simulink model "D2C_simulation_2boucles_0"  (R2013a)
settings: Solver=ode45  StartTime=0.0  StopTime=20  FixedStep=0.003  RelTol=1e-3
libraries: slctrlblks x2, simulink x2
settings Model: Creator=Propriétaire  LastModifiedBy=Propriétaire
settings DataIOCC: SignalLoggingSaveFormat=ModelDataLogs
settings OptimizationCC: ExpressionDepthLimit=2147483647
settings DebuggingCC: FcnCallInpInsideContextMsg=UseLocalSettings
settings GRTTargetCC: CombineOutputUpdateFcns=off  GRTInterface=on

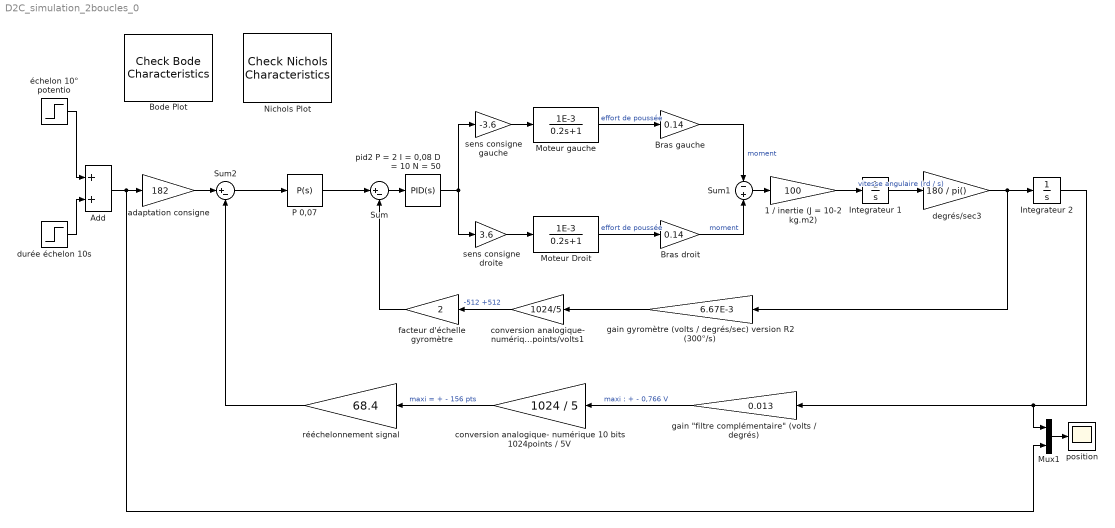
== system D2C_simulation_2boucles_0 ==
  1 / inertie (J = 10-2 kg.m2) : Gain  Gain=100
  Add : Sum
  Bode Plot : slctrlblks/Model Verification/Check Bode  Characteristics  InstantiateOnLoad=on  LinearizationIOs={'/Sum2', 1, 'in', 'on', '';'/rééchelonnement signal', 1, 'out', 'on', ''}  LinearizeAt=SnapshotTimes  SnapshotTimes=[0]  TriggerType=rising  SampleTime=auto  RateConversionMethod=zoh  PreWarpFreq=10  UseExactDelayModel=off  UseFullBlockNameLabels=off  UseBusSignalLabels=off  enabled=on  stopWhenAssertionFail=off  export=off  ViewDlgPos=[1323 39 510 390]  OpenViewOnLoad=on  LaunchViewOnOpen=on  FrequencyUnits=rad/s  MagnitudeUnits=dB  PhaseUnits=deg  TimeUnits=seconds  EnableUpperBound=off  UpperBoundFrequencies=[]  UpperBoundMagnitudes=[]  EnableLowerBound=off  LowerBoundFrequencies=[]  LowerBoundMagnitudes=[]
  Bras droit : Gain  Gain=0.14
  Bras gauche : Gain  Gain=0.14
  Integrateur 1 : Integrator
  Integrateur 2 : Integrator
  Moteur Droit : TransferFcn  Numerator=[1E-3]  Denominator=[0.2 1]
  Moteur gauche : TransferFcn  Numerator=[1E-3]  Denominator=[0.2 1]
  Mux1 : Mux  Inputs=2
  Nichols Plot : slctrlblks/Model Verification/Check Nichols Characteristics  InstantiateOnLoad=on  LinearizationIOs={'/Sum2', 1, 'in', 'on', '';'/rééchelonnement signal', 1, 'out', 'on', ''}  LinearizeAt=SnapshotTimes  SnapshotTimes=[0]  TriggerType=rising  SampleTime=auto  RateConversionMethod=zoh  PreWarpFreq=10  UseExactDelayModel=off  UseFullBlockNameLabels=off  UseBusSignalLabels=off  enabled=on  stopWhenAssertionFail=off  export=off  ViewDlgPos=[1322 516 510 390]  LaunchViewOnOpen=on  OpenViewOnLoad=on  FrequencyUnits=rad/s  MagnitudeUnits=dB  PhaseUnits=deg  TimeUnits=seconds  EnableMargins=off  GainMargin=[]  PhaseMargin=[]  EnableGainPhaseBound=off  GainPhaseBoundType={'upper'}  OLPhases=[]  OLGains=[]  EnableCLPeakGain=off  CLPeakGain=[]  FeedbackSign=-1
      settings: SaveToWorkspace=off  SaveName=sys
  P 0,07 : simulink/Continuous/PID Controller  Controller=P  TimeDomain=Continuous-time  SampleTime=1  IntegratorMethod=Forward Euler  FilterMethod=Forward Euler  Form=Parallel  P=0.07  I=5  D=0.0013  N=330  InitialConditionSource=internal  InitialConditionForIntegrator=0  InitialConditionForFilter=0  ExternalReset=none  LimitOutput=off  UpperSaturationLimit=inf  LowerSaturationLimit=-inf  LinearizeAsGain=off  AntiWindupMode=none  Kb=1  TrackingMode=off  Kt=1  PParamMin=[]  PParamMax=[]  IParamMin=[]  IParamMax=[]  DParamMin=[]  DParamMax=[]  NParamMin=[]  NParamMax=[]  KbParamMin=[]  KbParamMax=[]  KtParamMin=[]  KtParamMax=[]  POutMin=[]  POutMax=[]  IOutMin=[]  IOutMax=[]  DOutMin=[]  DOutMax=[]  NOutMin=[]  NOutMax=[]  KbOutMin=[]  KbOutMax=[]  KtOutMin=[]  KtOutMax=[]  IntegratorOutMin=[]  IntegratorOutMax=[]  FilterOutMin=[]  FilterOutMax=[]  SumOutMin=[]  SumOutMax=[]  SumI1OutMin=[]  SumI1OutMax=[]  SumI2OutMin=[]  SumI2OutMax=[]  SumI3OutMin=[]  SumI3OutMax=[]  SumDOutMin=[]  SumDOutMax=[]  SaturationOutMin=[]  SaturationOutMax=[]  IntegratorContinuousStateAttributes=''  IntegratorStateMustResolveToSignalObject=off  IntegratorRTWStateStorageClass=Auto  FilterContinuousStateAttributes=''  FilterStateMustResolveToSignalObject=off  FilterRTWStateStorageClass=Auto
  Sum : Sum  Inputs=|+-
  Sum1 : Sum  Inputs=-|+
  Sum2 : Sum  Inputs=|+-
  adaptation consigne : Gain  Gain=182
  conversion analogique- numérique points/volts1 : Gain  Gain=1024/5
  conversion analogique- numérique 10 bits 1024points / 5V : Gain  Gain=1024 / 5
  degrés/sec3 : Gain  Gain=180 / pi()
  durée échelon 10s : Step  Time=10  After=-10  SampleTime=0
  facteur d'échelle gyromètre : Gain  Gain=2
  "gain \"filtre complémentaire\" (volts / degrés)" : Gain  Gain=0.013
  gain gyromètre (volts / degrés/sec) version R2 (300°/s) : Gain  Gain=6.67E-3
  "pid2 P = 2 I = 0,08 D = 10 N = 50 " : simulink/Continuous/PID Controller  Controller=PID  TimeDomain=Continuous-time  SampleTime=1  IntegratorMethod=Forward Euler  FilterMethod=Forward Euler  Form=Parallel  P=2  I=0.08  D=10/50  N=50  InitialConditionSource=internal  InitialConditionForIntegrator=0  InitialConditionForFilter=0  ExternalReset=none  LimitOutput=off  UpperSaturationLimit=inf  LowerSaturationLimit=-inf  LinearizeAsGain=off  AntiWindupMode=none  Kb=1  TrackingMode=off  Kt=1  PParamMin=[]  PParamMax=[]  IParamMin=[]  IParamMax=[]  DParamMin=[]  DParamMax=[]  NParamMin=[]  NParamMax=[]  KbParamMin=[]  KbParamMax=[]  KtParamMin=[]  KtParamMax=[]  POutMin=[]  POutMax=[]  IOutMin=[]  IOutMax=[]  DOutMin=[]  DOutMax=[]  NOutMin=[]  NOutMax=[]  KbOutMin=[]  KbOutMax=[]  KtOutMin=[]  KtOutMax=[]  IntegratorOutMin=[]  IntegratorOutMax=[]  FilterOutMin=[]  FilterOutMax=[]  SumOutMin=[]  SumOutMax=[]  SumI1OutMin=[]  SumI1OutMax=[]  SumI2OutMin=[]  SumI2OutMax=[]  SumI3OutMin=[]  SumI3OutMax=[]  SumDOutMin=[]  SumDOutMax=[]  SaturationOutMin=[]  SaturationOutMax=[]  IntegratorContinuousStateAttributes=''  IntegratorStateMustResolveToSignalObject=off  IntegratorRTWStateStorageClass=Auto  FilterContinuousStateAttributes=''  FilterStateMustResolveToSignalObject=off  FilterRTWStateStorageClass=Auto
  position : Scope
      settings: YMin=-1  YMax=10
  rééchelonnement signal : Gain  Gain=68.4
  sens consigne droite : Gain  Gain=3.6
  sens consigne gauche : Gain  Gain=-3.6
  échelon 10° potentio : Step  Time=0  After=10  SampleTime=0
  wires:
  Moteur gauche/1 -> Bras gauche/1  "effort de poussée"
  Bras gauche/1 -> Sum1/1  "moment"
  Moteur Droit/1 -> Bras droit/1  "effort de poussée"
  Bras droit/1 -> Sum1/2  "moment"
  sens consigne gauche/1 -> Moteur gauche/1
  sens consigne droite/1 -> Moteur Droit/1
  Sum1/1 -> 1 / inertie (J = 10-2 kg.m2)/1
  gain gyromètre (volts / degrés/sec) version R2 (300°/s)/1 -> conversion analogique- numérique points/volts1/1
  1 / inertie (J = 10-2 kg.m2)/1 -> Integrateur 1/1
  Integrateur 1/1 -> degrés/sec3/1  "vitesse angulaire (rd / s)"
  Add/1 -> adaptation consigne/1, Mux1/2
  conversion analogique- numérique points/volts1/1 -> facteur d'échelle gyromètre/1  "-512 +512"
  "pid2 P = 2 I = 0,08 D = 10 N = 50 "/1 -> sens consigne droite/1, sens consigne gauche/1
  Mux1/1 -> position/1
  degrés/sec3/1 -> gain gyromètre (volts / degrés/sec) version R2 (300°/s)/1, Integrateur 2/1
  Integrateur 2/1 -> "gain \"filtre complémentaire\" (volts / degrés)"/1, Mux1/1
  "gain \"filtre complémentaire\" (volts / degrés)"/1 -> conversion analogique- numérique 10 bits 1024points / 5V/1  "maxi : + - 0,766 V"
  conversion analogique- numérique 10 bits 1024points / 5V/1 -> rééchelonnement signal/1  "maxi = + - 156 pts"
  adaptation consigne/1 -> Sum2/1
  Sum2/1 -> P 0,07/1
  facteur d'échelle gyromètre/1 -> Sum/2
  Sum/1 -> "pid2 P = 2 I = 0,08 D = 10 N = 50 "/1
  échelon 10° potentio/1 -> Add/1
  durée échelon 10s/1 -> Add/2
  rééchelonnement signal/1 -> Sum2/2
  P 0,07/1 -> Sum/1
